simulink subsystem "MotorDriveGear"  (R2024b)
settings: Solver=VariableStepAuto  StartTime=0.0  StopTime=10.0  RelTol=1e-3
model mask{max_torque=electricDrive.max_torque, max_power=electricDrive.max_power, Tctc=electricDrive.Tctc, motor_loss_map=electricDrive.motor_loss_map}
  mask prompts: Tctc "Motor torque control time constant(s)"
libraries: EmotorLib x1, sdl_lib x1
Description:
  | Motor Drive with Gear (No Thermal)
  | 
  | ⚡ Main Features:
  | - Electric motor with lumped electrical and mechanical dynamics
  | - Fixed gear for torque transmission to axle
  | - Motor input block: torque command, control, and battery signals
  | - No coolant or thermal dynamics (temperature fixed inputs)
  | - Emotor output provides torque, speed, and electrical power
  | - Internal signals: current, voltage, motor speed, and energy
  | 
  | 📤 Outputs: Motor Torque, Motor Speed, Electrical Power, Energy
  | 
  | 📌 Use Case: Fast simulations where thermal effects are not needed
settings Model: Creator=jjha  LastModifiedBy=jjha

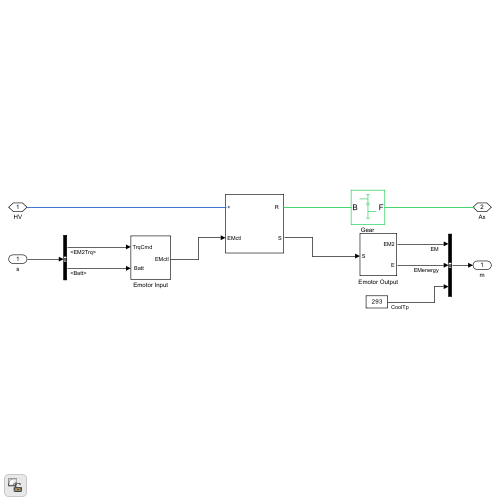
[thumbnail: Simulink's stored preview of the top-level diagram]
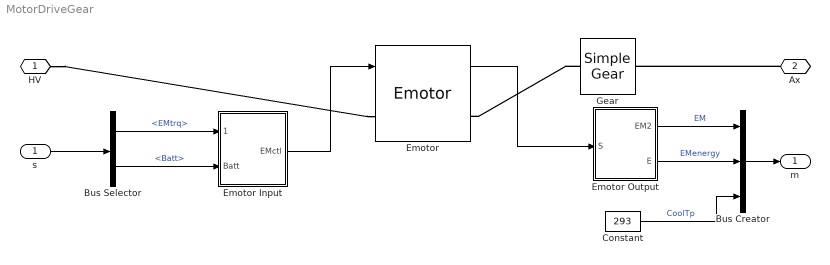
== system MotorDriveGear ==
  s : Inport
  Bus Creator : BusCreator  Inputs=3
  Bus Selector : BusSelector  OutputSignals=EMtrq,Batt
  Constant : Constant  Value=293
  Emotor : EmotorLib/Emotor  max_torque=electricDrive.max_torque  max_power=electricDrive.max_power  Tctc=electricDrive.Tctc  spMat=electricDrive.motor_loss_map.spMat  tqMat=electricDrive.motor_loss_map.tqMat  lossMat=electricDrive.motor_loss_map.lossMat
  Emotor Input : Subsystem
  Emotor Output : Subsystem
  Gear : sdl_lib/Gears/Simple Gear  ratio=10/3  rotation_direction=sdl.enum.shaftOutputDirection.same  friction_model=sdl.enum.gear_efficiencies_load.off  T_noload=0.1 N*m  T_nom=5 N*m  efficiency_nom=0.8  efficiency=0.8  temperature_TLU=[280, 300, 320] K  load_TLU=[1, 5, 10] N*m  efficiency_TLU=[.95, .9, .85]  efficiency_TLU2=[.85, .8, .75; .95, .9, .85; .85, .8, .7]  w_thr=0.01 rad/s  pwr_thr=0.001 W  enable_backlash=false  hardstop_model=simscape.enum.hardstop.smooth  backlash_distance=1e-3 mm  r_base=0.1 m  transition=1e-4 mm  backlash_stiffness=1e7 N/m  backlash_damping=1e6 N*s/m  coeff_rest=0  v_tol=0.001 m/s  f_tol=0 N  mu_visc=[0, 0] N*m*s/rad  thermal_mass=50 J/K  temperature_specify=off  temperature_priority=High  temperature=300 K  temperature_nominal_specify=off  temperature_nominal_value=1  temperature_nominal_unit=K  x_backlash_specify=off  x_backlash_priority=None  x_backlash=0 mm  x_backlash_nominal_specify=off  x_backlash_nominal_value=1  x_backlash_nominal_unit=mm  f_hardstop_specify=off  f_hardstop_priority=None  f_hardstop=0 N  f_hardstop_nominal_specify=off  f_hardstop_nominal_value=1  f_hardstop_nominal_unit=N  v_backlash_specify=off  v_backlash_priority=None  v_backlash=0 m/s  v_backlash_nominal_specify=off  v_backlash_nominal_value=1  v_backlash_nominal_unit=m/s
  HV : PMIOPort  Side=Left
  Ax : PMIOPort  Port=2  Side=Right
  m : Outport
  wires:
  Bus Selector/1 -> Emotor Input/1(TrqCmd)  "<EMtrq>"
  Bus Selector/2 -> Emotor Input/2(" Batt")  "<Batt>"
  Emotor/1 -> Emotor Output/1(S)
  Emotor Input/1(EMctl) -> Emotor/1
  Bus Creator/1 -> m/1
  Emotor Output/1(EM2) -> Bus Creator/1  "EM"
  Emotor Output/2(E) -> Bus Creator/2  "EMenergy"
  s/1 -> Bus Selector/1
  Constant/1 -> Bus Creator/3  "CoolTp"
  connections:
  Gear/LConn1 -- Emotor/RConn1
  Ax/RConn1 -- Gear/RConn1
  HV/RConn1 -- Emotor/LConn1

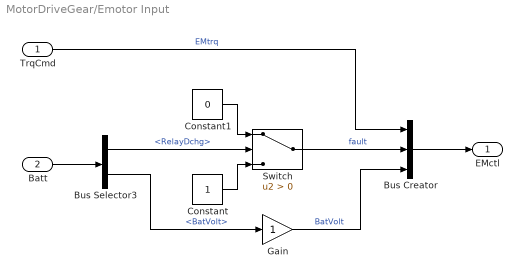
== system MotorDriveGear/Emotor Input ==
  TrqCmd : Inport
  " Batt" : Inport  Port=2
  Bus Creator : BusCreator  Inputs=3
  Bus Selector3 : BusSelector  OutputSignals=Relay.RelayDchg,BattSensor.BatVolt
  Constant : Constant
  Constant1 : Constant  Value=0
  Gain : Gain
  Switch : Switch  Criteria=u2 > Threshold  SaturateOnIntegerOverflow=off  InputSameDT=off
  EMctl : Outport
  wires:
  Gain/1 -> Bus Creator/3  "BatVolt"
  Bus Selector3/2 -> Gain/1  "<BatVolt>"
  Bus Creator/1 -> EMctl/1
  " Batt"/1 -> Bus Selector3/1
  Bus Selector3/1 -> Switch/2  "<RelayDchg>"
  Constant/1 -> Switch/3
  Constant1/1 -> Switch/1
  Switch/1 -> Bus Creator/2  "fault"
  TrqCmd/1 -> Bus Creator/1  "EMtrq"

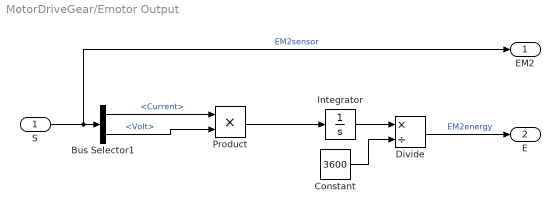
== system MotorDriveGear/Emotor Output ==
  S : Inport
  Bus Selector1 : BusSelector  OutputSignals=Current,Volt
  Constant : Constant  Value=3600
  Divide : Product  Inputs=*/
  Integrator : Integrator
  Product : Product
  EM2 : Outport
  E : Outport  Port=2
  wires:
  Bus Selector1/1 -> Product/1  "<Current>"
  Bus Selector1/2 -> Product/2  "<Volt>"
  S/1 -> Bus Selector1/1, EM2/1  "EM2sensor"
  Product/1 -> Integrator/1
  Integrator/1 -> Divide/1
  Constant/1 -> Divide/2
  Divide/1 -> E/1  "EM2energy"
